simulink model "ControlSystem"  (R2021b)
settings: Solver=VariableStepAuto  StartTime=simIn(1,1)  StopTime=simIn(end,1)  RelTol=1e-3
values from neighbouring files (symbols this model uses):
  A = -inv(L)*R    [PlasmalessModel.m]
  B = L\S    [PlasmalessModel.m]
  C = eye(circuitNumber,length(A))    [PlasmalessModel.m]
  Controller = struct('R1',pid(Rcontr(1,1)),'R2',pid(Rcontr(2,2)),'R3',pid(Rcontr(3,3)),'R4',pid(Rcontr(4,4)),'R5',      pid(Rcontr(5,5)),'R6',pid(Rcontr(6,6)),'R7',pid(Rcontr(7,7)),'R8',pid(Rcontr(8,8)),'R9',pid(Rcontr(9,9)),'R10',      pid(Rcontr(10,10)),'R11',pid(Rcontr(11,11)),'R12',pid(Rcontr(12,12)))    [GeneticAlgorithm.m]    (also in OptimalTunedGA.mat = ; PIDController.m = struct('R1',R1,'R2',R2,'R3',R3,'R4',R4,'R5',R5,'R6',R6,     ; RLocusController.m = struct('R1',R1,'R2',R2,'R3',R3,'R4',R4,'R5',R5,'R6',R6,     )
  D = zeros(circuitNumber,circuitNumber)    [PlasmalessModel.m]
  dt = 0.001    [GeneticAlgorithm.m]    (also in PlasmalessModel.m; ReferenceDatabase.m)
  fil1 = zpk(minreal(R1 - k1 - r1(end)/s, 1e-2))    [RLocusController.m]
  fil10 = zpk(minreal(R10 - k10 - r10(end)/s, 1e-2))    [RLocusController.m]
  fil11 = zpk(minreal(R11 - k11 - r11(end)/s, 1e-2))    [RLocusController.m]
  fil12 = zpk(minreal(R12 - k12 - r12(end)/s, 1e-2))    [RLocusController.m]
  fil2 = zpk(minreal(R2 - k2 - r2(end)/s, 1e-2))    [RLocusController.m]
  fil3 = zpk(minreal(R3 - k3 - r3(end)/s, 1e-2))    [RLocusController.m]
  fil4 = zpk(minreal(R4 - k4 - r4(end)/s, 1e-2))    [RLocusController.m]
  fil5 = zpk(minreal(R5 - k5 - r5(end)/s, 1e-2))    [RLocusController.m]
  fil6 = zpk(minreal(R6 - k6 - r6(end)/s, 1e-2))    [RLocusController.m]
  fil7 = zpk(minreal(R7 - k7 - r7(end)/s, 1e-2))    [RLocusController.m]
  fil8 = zpk(minreal(R8 - k8 - r8(end)/s, 1e-2))    [RLocusController.m]
  fil9 = zpk(minreal(R9 - k9 - r9(end)/s, 1e-2))    [RLocusController.m]
  PSdelay = 1.67e-3    (= 0.00167)    [PlasmalessModel.m]
  PSden = [7e-3 1]    [PlasmalessModel.m]
  PSnum = 1    [PlasmalessModel.m]
  PSsat = [350 350 350 350 350 350           800 800 400 400 330 330]    [PlasmalessModel.m]
  sys1 = balred(sys(1,1),ord)    [PlasmalessModel.m]
  sys10 = balred(sys(10,10),ord)    [PlasmalessModel.m]
  sys11 = balred(sys(11,11),ord)    [PlasmalessModel.m]
  sys12 = balred(sys(12,12),ord)    [PlasmalessModel.m]
  sys2 = balred(sys(2,2),ord)    [PlasmalessModel.m]
  sys3 = balred(sys(3,3),ord)    [PlasmalessModel.m]
  sys4 = balred(sys(4,4),ord)    [PlasmalessModel.m]
  sys5 = balred(sys(5,5),ord)    [PlasmalessModel.m]
  sys6 = balred(sys(6,6),ord)    [PlasmalessModel.m]
  sys7 = balred(sys(7,7),ord)    [PlasmalessModel.m]
  sys8 = balred(sys(8,8),ord)    [PlasmalessModel.m]
  sys9 = balred(sys(9,9),ord)    [PlasmalessModel.m]
  varIpf = Scenario.Reference4.var    [PlasmalessModel.m]    (also in ReferenceDatabase.m)
undefined symbols (not defined in the file or in its folder): k1, k10, k11, k12, k2, k3, k4, k5, k6, k7, k8, k9
libraries: simulink x98, cstblocks x60
(part 2 of 4)

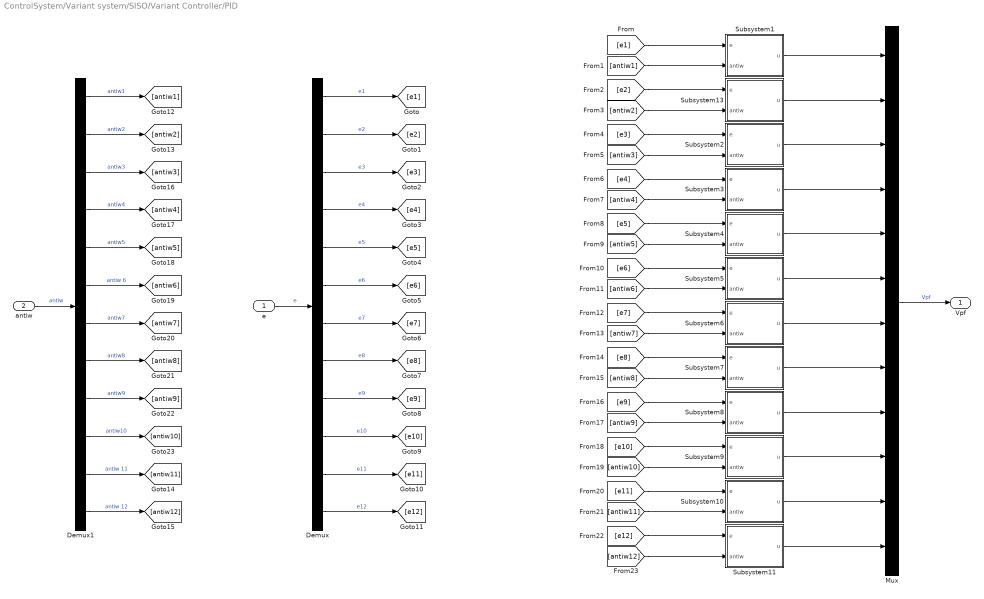
== system ControlSystem/Variant system/SISO/Variant Controller/PID ==
  e : Inport
  antiw : Inport  Port=2
  Demux : Demux  Outputs=12
  Demux1 : Demux  Outputs=12
  Mux : Mux  Inputs=12
  Subsystem1 : Subsystem  mask(Custom PID){Ki=Controller.R1.Ki, Kp=Controller.R1.Kp, Kd=Controller.R1.Kd, Tf=[Controller.R1.Tf 1], Threshold=PSsat(1)}
      mask prompts: Ki "Integral Gain"; Kp "Proportional Gain"; Kd "Derivative Gain"; Tf "Filtered Derivative"
      mask TypeOptions Ki: Integral Gain/Gain
      mask TypeOptions Kp: Proportional Gain/Gain
      mask TypeOptions Kd: Derivative Gain/Gain
      mask TypeOptions Tf: Filtered Derivative/Denominator
      mask TypeOptions Threshold:
      | Clamping/Compare
      | To Threshold/const
      mask DialogControl Container1 Prompt: Gain and Compensator
      mask DialogControl Container2 Prompt: Anti Windup
  Subsystem10 : Subsystem  mask(Custom PID){Ki=Controller.R11.Ki, Kp=Controller.R11.Kp, Kd=Controller.R11.Kd, Tf=[Controller.R11.Tf 1], Threshold=PSsat(11)}
      mask prompts: Ki "Integral Gain"; Kp "Proportional Gain"; Kd "Derivative Gain"; Tf "Filtered Derivative"
      mask TypeOptions Ki: Integral Gain/Gain
      mask TypeOptions Kp: Proportional Gain/Gain
      mask TypeOptions Kd: Derivative Gain/Gain
      mask TypeOptions Tf: Filtered Derivative/Denominator
      mask TypeOptions Threshold:
      | Clamping/Compare
      | To Threshold/const
      mask DialogControl Container1 Prompt: Gain and Compensator
      mask DialogControl Container2 Prompt: Anti Windup
  Subsystem11 : Subsystem  mask(Custom PID){Ki=Controller.R12.Ki, Kp=Controller.R12.Kp, Kd=Controller.R12.Kd, Tf=[Controller.R12.Tf 1], Threshold=PSsat(12)}
      mask prompts: Ki "Integral Gain"; Kp "Proportional Gain"; Kd "Derivative Gain"; Tf "Filtered Derivative"
      mask TypeOptions Ki: Integral Gain/Gain
      mask TypeOptions Kp: Proportional Gain/Gain
      mask TypeOptions Kd: Derivative Gain/Gain
      mask TypeOptions Tf: Filtered Derivative/Denominator
      mask TypeOptions Threshold:
      | Clamping/Compare
      | To Threshold/const
      mask DialogControl Container1 Prompt: Gain and Compensator
      mask DialogControl Container2 Prompt: Anti Windup
  Subsystem13 : Subsystem  mask(Custom PID){Ki=Controller.R2.Ki, Kp=Controller.R2.Kp, Kd=Controller.R2.Kd, Tf=[Controller.R2.Tf 1], Threshold=PSsat(2)}
      mask prompts: Ki "Integral Gain"; Kp "Proportional Gain"; Kd "Derivative Gain"; Tf "Filtered Derivative"
      mask TypeOptions Ki: Integral Gain/Gain
      mask TypeOptions Kp: Proportional Gain/Gain
      mask TypeOptions Kd: Derivative Gain/Gain
      mask TypeOptions Tf: Filtered Derivative/Denominator
      mask TypeOptions Threshold:
      | Clamping/Compare
      | To Threshold/const
      mask DialogControl Container1 Prompt: Gain and Compensator
      mask DialogControl Container2 Prompt: Anti Windup
  Subsystem2 : Subsystem  mask(Custom PID){Ki=Controller.R3.Ki, Kp=Controller.R3.Kp, Kd=Controller.R3.Kd, Tf=[Controller.R3.Tf 1], Threshold=PSsat(3)}
      mask prompts: Ki "Integral Gain"; Kp "Proportional Gain"; Kd "Derivative Gain"; Tf "Filtered Derivative"
      mask TypeOptions Ki: Integral Gain/Gain
      mask TypeOptions Kp: Proportional Gain/Gain
      mask TypeOptions Kd: Derivative Gain/Gain
      mask TypeOptions Tf: Filtered Derivative/Denominator
      mask TypeOptions Threshold:
      | Clamping/Compare
      | To Threshold/const
      mask DialogControl Container1 Prompt: Gain and Compensator
      mask DialogControl Container2 Prompt: Anti Windup
  Subsystem3 : Subsystem  mask(Custom PID){Ki=Controller.R4.Ki, Kp=Controller.R4.Kp, Kd=Controller.R4.Kd, Tf=[Controller.R4.Tf 1], Threshold=PSsat(4)}
      mask prompts: Ki "Integral Gain"; Kp "Proportional Gain"; Kd "Derivative Gain"; Tf "Filtered Derivative"
      mask TypeOptions Ki: Integral Gain/Gain
      mask TypeOptions Kp: Proportional Gain/Gain
      mask TypeOptions Kd: Derivative Gain/Gain
      mask TypeOptions Tf: Filtered Derivative/Denominator
      mask TypeOptions Threshold:
      | Clamping/Compare
      | To Threshold/const
      mask DialogControl Container1 Prompt: Gain and Compensator
      mask DialogControl Container2 Prompt: Anti Windup
  Subsystem4 : Subsystem  mask(Custom PID){Ki=Controller.R5.Ki, Kp=Controller.R5.Kp, Kd=Controller.R5.Kd, Tf=[Controller.R5.Tf 1], Threshold=PSsat(5)}
      mask prompts: Ki "Integral Gain"; Kp "Proportional Gain"; Kd "Derivative Gain"; Tf "Filtered Derivative"
      mask TypeOptions Ki: Integral Gain/Gain
      mask TypeOptions Kp: Proportional Gain/Gain
      mask TypeOptions Kd: Derivative Gain/Gain
      mask TypeOptions Tf: Filtered Derivative/Denominator
      mask TypeOptions Threshold:
      | Clamping/Compare
      | To Threshold/const
      mask DialogControl Container1 Prompt: Gain and Compensator
      mask DialogControl Container2 Prompt: Anti Windup
  Subsystem5 : Subsystem  mask(Custom PID){Ki=Controller.R6.Ki, Kp=Controller.R6.Kp, Kd=Controller.R6.Kd, Tf=[Controller.R6.Tf 1], Threshold=PSsat(6)}
      mask prompts: Ki "Integral Gain"; Kp "Proportional Gain"; Kd "Derivative Gain"; Tf "Filtered Derivative"
      mask TypeOptions Ki: Integral Gain/Gain
      mask TypeOptions Kp: Proportional Gain/Gain
      mask TypeOptions Kd: Derivative Gain/Gain
      mask TypeOptions Tf: Filtered Derivative/Denominator
      mask TypeOptions Threshold:
      | Clamping/Compare
      | To Threshold/const
      mask DialogControl Container1 Prompt: Gain and Compensator
      mask DialogControl Container2 Prompt: Anti Windup
  Subsystem6 : Subsystem  mask(Custom PID){Ki=Controller.R7.Ki, Kp=Controller.R7.Kp, Kd=Controller.R7.Kd, Tf=[Controller.R7.Tf 1], Threshold=PSsat(7)}
      mask prompts: Ki "Integral Gain"; Kp "Proportional Gain"; Kd "Derivative Gain"; Tf "Filtered Derivative"
      mask TypeOptions Ki: Integral Gain/Gain
      mask TypeOptions Kp: Proportional Gain/Gain
      mask TypeOptions Kd: Derivative Gain/Gain
      mask TypeOptions Tf: Filtered Derivative/Denominator
      mask TypeOptions Threshold:
      | Clamping/Compare
      | To Threshold/const
      mask DialogControl Container1 Prompt: Gain and Compensator
      mask DialogControl Container2 Prompt: Anti Windup
  Subsystem7 : Subsystem  mask(Custom PID){Ki=Controller.R8.Ki, Kp=Controller.R8.Kp, Kd=Controller.R8.Kd, Tf=[Controller.R8.Tf 1], Threshold=PSsat(8)}
      mask prompts: Ki "Integral Gain"; Kp "Proportional Gain"; Kd "Derivative Gain"; Tf "Filtered Derivative"
      mask TypeOptions Ki: Integral Gain/Gain
      mask TypeOptions Kp: Proportional Gain/Gain
      mask TypeOptions Kd: Derivative Gain/Gain
      mask TypeOptions Tf: Filtered Derivative/Denominator
      mask TypeOptions Threshold:
      | Clamping/Compare
      | To Threshold/const
      mask DialogControl Container1 Prompt: Gain and Compensator
      mask DialogControl Container2 Prompt: Anti Windup
  Subsystem8 : Subsystem  mask(Custom PID){Ki=Controller.R9.Ki, Kp=Controller.R9.Kp, Kd=Controller.R9.Kd, Tf=[Controller.R9.Tf 1], Threshold=PSsat(9)}
      mask prompts: Ki "Integral Gain"; Kp "Proportional Gain"; Kd "Derivative Gain"; Tf "Filtered Derivative"
      mask TypeOptions Ki: Integral Gain/Gain
      mask TypeOptions Kp: Proportional Gain/Gain
      mask TypeOptions Kd: Derivative Gain/Gain
      mask TypeOptions Tf: Filtered Derivative/Denominator
      mask TypeOptions Threshold:
      | Clamping/Compare
      | To Threshold/const
      mask DialogControl Container1 Prompt: Gain and Compensator
      mask DialogControl Container2 Prompt: Anti Windup
  Subsystem9 : Subsystem  mask(Custom PID){Ki=Controller.R10.Ki, Kp=Controller.R10.Kp, Kd=Controller.R10.Kd, Tf=[Controller.R10.Tf 1], Threshold=PSsat(10)}
      mask prompts: Ki "Integral Gain"; Kp "Proportional Gain"; Kd "Derivative Gain"; Tf "Filtered Derivative"
      mask TypeOptions Ki: Integral Gain/Gain
      mask TypeOptions Kp: Proportional Gain/Gain
      mask TypeOptions Kd: Derivative Gain/Gain
      mask TypeOptions Tf: Filtered Derivative/Denominator
      mask TypeOptions Threshold:
      | Clamping/Compare
      | To Threshold/const
      mask DialogControl Container1 Prompt: Gain and Compensator
      mask DialogControl Container2 Prompt: Anti Windup
  Vpf : Outport
  wires:
  Subsystem10/1(u) -> Mux/11
  e/1 -> Demux/1  "e"
  [antiw3] -> Subsystem2/2(antiw)
  Demux/1 -> [e1]  "e1"
  [e1] -> Subsystem1/1(e)
  Demux1/7 -> [antiw7]  "antiw7"
  Demux/2 -> [e2]  "e2"
  Demux/12 -> [e12]  "e12"
  Subsystem8/1(u) -> Mux/9
  Demux/3 -> [e3]  "e3"
  Demux/8 -> [e8]  "e8"
  Demux/9 -> [e9]  "e9"
  Demux1/2 -> [antiw2]  "antiw2"
  Demux/7 -> [e7]  "e7"
  Demux1/1 -> [antiw1]  "antiw1"
  Demux/11 -> [e11]  "e11"
  Demux1/5 -> [antiw5]  "antiw5"
  [e6] -> Subsystem5/1(e)
  [antiw7] -> Subsystem6/2(antiw)
  [e11] -> Subsystem10/1(e)
  [e5] -> Subsystem4/1(e)
  [e12] -> Subsystem11/1(e)
  Demux1/10 -> [antiw10]  "antiw10"
  [antiw4] -> Subsystem3/2(antiw)
  Demux1/8 -> [antiw8]  "antiw8"
  [antiw6] -> Subsystem5/2(antiw)
  [e10] -> Subsystem9/1(e)
  [antiw11] -> Subsystem10/2(antiw)
  antiw/1 -> Demux1/1  "antiw"
  Demux/6 -> [e6]  "e6"
  Demux1/11 -> [antiw11]  "antiw 11"
  [e3] -> Subsystem2/1(e)
  Demux1/6 -> [antiw6]  "antiw 6"
  Demux1/3 -> [antiw3]  "antiw3"
  Demux1/12 -> [antiw12]  "antiw 12"
  [e9] -> Subsystem8/1(e)
  [antiw2] -> Subsystem13/2(antiw)
  Demux1/9 -> [antiw9]  "antiw9"
  [antiw10] -> Subsystem9/2(antiw)
  [antiw8] -> Subsystem7/2(antiw)
  Subsystem3/1(u) -> Mux/4
  Demux/10 -> [e10]  "e10"
  Demux/5 -> [e5]  "e5"
  Subsystem2/1(u) -> Mux/3
  Demux/4 -> [e4]  "e4"
  Subsystem5/1(u) -> Mux/6
  [antiw9] -> Subsystem8/2(antiw)
  Subsystem1/1(u) -> Mux/1
  Mux/1 -> Vpf/1  "Vpf"
  Subsystem11/1(u) -> Mux/12
  [antiw1] -> Subsystem1/2(antiw)
  [antiw5] -> Subsystem4/2(antiw)
  [antiw12] -> Subsystem11/2(antiw)
  [e7] -> Subsystem6/1(e)
  Subsystem13/1(u) -> Mux/2
  [e4] -> Subsystem3/1(e)
  Demux1/4 -> [antiw4]  "antiw4"
  [e8] -> Subsystem7/1(e)
  Subsystem6/1(u) -> Mux/7
  Subsystem7/1(u) -> Mux/8
  Subsystem9/1(u) -> Mux/10
  Subsystem4/1(u) -> Mux/5
  [e2] -> Subsystem13/1(e)

== system ControlSystem/Variant system/SISO/Variant Controller/RlocusNOantiwindup ==
  e : Inport
  Demux : Demux  Outputs=12
  LTI System : cstblocks/LTI System  sys=R1  IC=[]
  LTI System1 : cstblocks/LTI System  sys=R2  IC=[]
  LTI System10 : cstblocks/LTI System  sys=R11  IC=[]
  LTI System11 : cstblocks/LTI System  sys=R12  IC=[]
  LTI System2 : cstblocks/LTI System  sys=R3  IC=[]
  LTI System3 : cstblocks/LTI System  sys=R4  IC=[]
  LTI System4 : cstblocks/LTI System  sys=R5  IC=[]
  LTI System5 : cstblocks/LTI System  sys=R6  IC=[]
  LTI System6 : cstblocks/LTI System  sys=R7  IC=[]
  LTI System7 : cstblocks/LTI System  sys=R8  IC=[]
  LTI System8 : cstblocks/LTI System  sys=R9  IC=[]
  LTI System9 : cstblocks/LTI System  sys=R10  IC=[]
  Mux : Mux  Inputs=12
  Vpf : Outport
  wires:
  LTI System11/1 -> Mux/12
  LTI System1/1 -> Mux/2
  LTI System5/1 -> Mux/6
  LTI System7/1 -> Mux/8
  Demux/10 -> LTI System9/1
  Demux/8 -> LTI System7/1
  Demux/7 -> LTI System6/1
  Demux/6 -> LTI System5/1
  LTI System/1 -> Mux/1
  Demux/12 -> LTI System11/1
  Demux/3 -> LTI System2/1
  Demux/1 -> LTI System/1
  LTI System2/1 -> Mux/3
  Demux/4 -> LTI System3/1
  LTI System4/1 -> Mux/5
  Demux/2 -> LTI System1/1
  Demux/9 -> LTI System8/1
  Demux/5 -> LTI System4/1
  LTI System3/1 -> Mux/4
  LTI System10/1 -> Mux/11
  LTI System6/1 -> Mux/7
  e/1 -> Demux/1  "e"
  Mux/1 -> Vpf/1  "Vpf"
  LTI System8/1 -> Mux/9
  LTI System9/1 -> Mux/10
  Demux/11 -> LTI System10/1

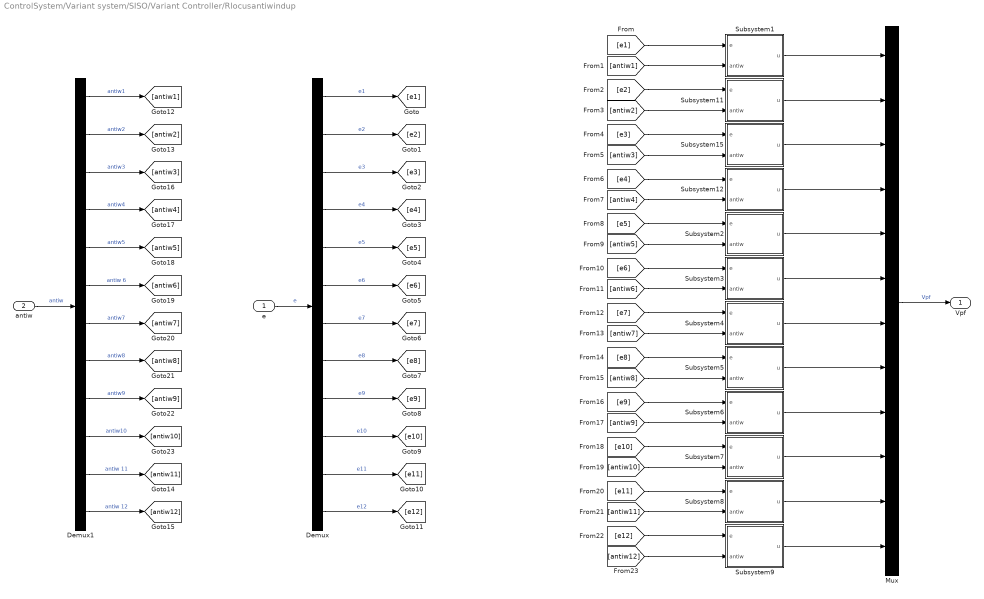
== system ControlSystem/Variant system/SISO/Variant Controller/Rlocusantiwindup ==
  e : Inport
  antiw : Inport  Port=2
  Demux : Demux  Outputs=12
  Demux1 : Demux  Outputs=12
  Mux : Mux  Inputs=12
  Subsystem1 : Subsystem  mask(Fractal Transfer Function){Ki=r1(end), Kp=k1, Compensator=fil1, Threshold=PSsat(1)}
      mask prompts: Ki "Integral Gain"; Kp "Proportional Gain"
      mask help: Fractal Transfer Function of a controller in a general rational transfer function form. The controller is decomposed in an Integral term, a Proportional term and a compensator.
      mask TypeOptions Ki: Integral Gain/Gain
      mask TypeOptions Kp: Proportional Gain/Gain
      mask TypeOptions Compensator: ZPK compensator/sys
      mask TypeOptions Threshold:
      | Clamping/Compare
      | To Threshold/const
      mask DialogControl Container1 Prompt: Gain and Compensator
      mask DialogControl Container2 Prompt: Anti Windup
  Subsystem11 : Subsystem  mask(Fractal Transfer Function){Ki=r2(end), Kp=k2, Compensator=fil2, Threshold=PSsat(2)}
      mask prompts: Ki "Integral Gain"; Kp "Proportional Gain"
      mask help: Fractal Transfer Function of a controller in a general rational transfer function form. The controller is decomposed in an Integral term, a Proportional term and a compensator.
      mask TypeOptions Ki: Integral Gain/Gain
      mask TypeOptions Kp: Proportional Gain/Gain
      mask TypeOptions Compensator: ZPK compensator/sys
      mask TypeOptions Threshold:
      | Clamping/Compare
      | To Threshold/const
      mask DialogControl Container1 Prompt: Gain and Compensator
      mask DialogControl Container2 Prompt: Anti Windup
  Subsystem12 : Subsystem  mask(Fractal Transfer Function){Ki=r4(end), Kp=k4, Compensator=fil4, Threshold=PSsat(4)}
      mask prompts: Ki "Integral Gain"; Kp "Proportional Gain"
      mask help: Fractal Transfer Function of a controller in a general rational transfer function form. The controller is decomposed in an Integral term, a Proportional term and a compensator.
      mask TypeOptions Ki: Integral Gain/Gain
      mask TypeOptions Kp: Proportional Gain/Gain
      mask TypeOptions Compensator: ZPK compensator/sys
      mask TypeOptions Threshold:
      | Clamping/Compare
      | To Threshold/const
      mask DialogControl Container1 Prompt: Gain and Compensator
      mask DialogControl Container2 Prompt: Anti Windup
  Subsystem15 : Subsystem  mask(Fractal Transfer Function){Ki=r3(end), Kp=k3, Compensator=fil3, Threshold=PSsat(3)}
      mask prompts: Ki "Integral Gain"; Kp "Proportional Gain"
      mask help: Fractal Transfer Function of a controller in a general rational transfer function form. The controller is decomposed in an Integral term, a Proportional term and a compensator.
      mask TypeOptions Ki: Integral Gain/Gain
      mask TypeOptions Kp: Proportional Gain/Gain
      mask TypeOptions Compensator: ZPK compensator/sys
      mask TypeOptions Threshold:
      | Clamping/Compare
      | To Threshold/const
      mask DialogControl Container1 Prompt: Gain and Compensator
      mask DialogControl Container2 Prompt: Anti Windup
  Subsystem2 : Subsystem  mask(Fractal Transfer Function){Ki=r5(end), Kp=k5, Compensator=fil5, Threshold=PSsat(5)}
      mask prompts: Ki "Integral Gain"; Kp "Proportional Gain"
      mask help: Fractal Transfer Function of a controller in a general rational transfer function form. The controller is decomposed in an Integral term, a Proportional term and a compensator.
      mask TypeOptions Ki: Integral Gain/Gain
      mask TypeOptions Kp: Proportional Gain/Gain
      mask TypeOptions Compensator: ZPK compensator/sys
      mask TypeOptions Threshold:
      | Clamping/Compare
      | To Threshold/const
      mask DialogControl Container1 Prompt: Gain and Compensator
      mask DialogControl Container2 Prompt: Anti Windup
  Subsystem3 : Subsystem  mask(Fractal Transfer Function){Ki=r6(end), Kp=k6, Compensator=fil6, Threshold=PSsat(6)}
      mask prompts: Ki "Integral Gain"; Kp "Proportional Gain"
      mask help: Fractal Transfer Function of a controller in a general rational transfer function form. The controller is decomposed in an Integral term, a Proportional term and a compensator.
      mask TypeOptions Ki: Integral Gain/Gain
      mask TypeOptions Kp: Proportional Gain/Gain
      mask TypeOptions Compensator: ZPK compensator/sys
      mask TypeOptions Threshold:
      | Clamping/Compare
      | To Threshold/const
      mask DialogControl Container1 Prompt: Gain and Compensator
      mask DialogControl Container2 Prompt: Anti Windup
  Subsystem4 : Subsystem  mask(Fractal Transfer Function){Ki=r7(end), Kp=k7, Compensator=fil7, Threshold=PSsat(7)}
      mask prompts: Ki "Integral Gain"; Kp "Proportional Gain"
      mask help: Fractal Transfer Function of a controller in a general rational transfer function form. The controller is decomposed in an Integral term, a Proportional term and a compensator.
      mask TypeOptions Ki: Integral Gain/Gain
      mask TypeOptions Kp: Proportional Gain/Gain
      mask TypeOptions Compensator: ZPK compensator/sys
      mask TypeOptions Threshold:
      | Clamping/Compare
      | To Threshold/const
      mask DialogControl Container1 Prompt: Gain and Compensator
      mask DialogControl Container2 Prompt: Anti Windup
  Subsystem5 : Subsystem  mask(Fractal Transfer Function){Ki=r8(end), Kp=k8, Compensator=fil8, Threshold=PSsat(8)}
      mask prompts: Ki "Integral Gain"; Kp "Proportional Gain"
      mask help: Fractal Transfer Function of a controller in a general rational transfer function form. The controller is decomposed in an Integral term, a Proportional term and a compensator.
      mask TypeOptions Ki: Integral Gain/Gain
      mask TypeOptions Kp: Proportional Gain/Gain
      mask TypeOptions Compensator: ZPK compensator/sys
      mask TypeOptions Threshold:
      | Clamping/Compare
      | To Threshold/const
      mask DialogControl Container1 Prompt: Gain and Compensator
      mask DialogControl Container2 Prompt: Anti Windup
  Subsystem6 : Subsystem  mask(Fractal Transfer Function){Ki=r9(end), Kp=k9, Compensator=fil9, Threshold=PSsat(9)}
      mask prompts: Ki "Integral Gain"; Kp "Proportional Gain"
      mask help: Fractal Transfer Function of a controller in a general rational transfer function form. The controller is decomposed in an Integral term, a Proportional term and a compensator.
      mask TypeOptions Ki: Integral Gain/Gain
      mask TypeOptions Kp: Proportional Gain/Gain
      mask TypeOptions Compensator: ZPK compensator/sys
      mask TypeOptions Threshold:
      | Clamping/Compare
      | To Threshold/const
      mask DialogControl Container1 Prompt: Gain and Compensator
      mask DialogControl Container2 Prompt: Anti Windup
  Subsystem7 : Subsystem  mask(Fractal Transfer Function){Ki=r10(end), Kp=k10, Compensator=fil10, Threshold=PSsat(10)}
      mask prompts: Ki "Integral Gain"; Kp "Proportional Gain"
      mask help: Fractal Transfer Function of a controller in a general rational transfer function form. The controller is decomposed in an Integral term, a Proportional term and a compensator.
      mask TypeOptions Ki: Integral Gain/Gain
      mask TypeOptions Kp: Proportional Gain/Gain
      mask TypeOptions Compensator: ZPK compensator/sys
      mask TypeOptions Threshold:
      | Clamping/Compare
      | To Threshold/const
      mask DialogControl Container1 Prompt: Gain and Compensator
      mask DialogControl Container2 Prompt: Anti Windup
  Subsystem8 : Subsystem  mask(Fractal Transfer Function){Ki=r11(end), Kp=k11, Compensator=fil11, Threshold=PSsat(11)}
      mask prompts: Ki "Integral Gain"; Kp "Proportional Gain"
      mask help: Fractal Transfer Function of a controller in a general rational transfer function form. The controller is decomposed in an Integral term, a Proportional term and a compensator.
      mask TypeOptions Ki: Integral Gain/Gain
      mask TypeOptions Kp: Proportional Gain/Gain
      mask TypeOptions Compensator: ZPK compensator/sys
      mask TypeOptions Threshold:
      | Clamping/Compare
      | To Threshold/const
      mask DialogControl Container1 Prompt: Gain and Compensator
      mask DialogControl Container2 Prompt: Anti Windup
  Subsystem9 : Subsystem  mask(Fractal Transfer Function){Ki=r12(end), Kp=k12, Compensator=fil12, Threshold=PSsat(12)}
      mask prompts: Ki "Integral Gain"; Kp "Proportional Gain"
      mask help: Fractal Transfer Function of a controller in a general rational transfer function form. The controller is decomposed in an Integral term, a Proportional term and a compensator.
      mask TypeOptions Ki: Integral Gain/Gain
      mask TypeOptions Kp: Proportional Gain/Gain
      mask TypeOptions Compensator: ZPK compensator/sys
      mask TypeOptions Threshold:
      | Clamping/Compare
      | To Threshold/const
      mask DialogControl Container1 Prompt: Gain and Compensator
      mask DialogControl Container2 Prompt: Anti Windup
  Vpf : Outport
  wires:
  [e2] -> Subsystem11/1(e)
  Subsystem2/1(u) -> Mux/5
  Subsystem7/1(u) -> Mux/10
  Subsystem5/1(u) -> Mux/8
  Subsystem4/1(u) -> Mux/7
  [e8] -> Subsystem5/1(e)
  Demux1/4 -> [antiw4]  "antiw4"
  [e4] -> Subsystem12/1(e)
  Subsystem11/1(u) -> Mux/2
  [e7] -> Subsystem4/1(e)
  [antiw12] -> Subsystem9/2(antiw)
  [antiw5] -> Subsystem2/2(antiw)
  [antiw1] -> Subsystem1/2(antiw)
  Subsystem9/1(u) -> Mux/12
  Mux/1 -> Vpf/1  "Vpf"
  Subsystem1/1(u) -> Mux/1
  [antiw9] -> Subsystem6/2(antiw)
  Subsystem3/1(u) -> Mux/6
  Demux/4 -> [e4]  "e4"
  Subsystem15/1(u) -> Mux/3
  Demux/5 -> [e5]  "e5"
  Demux/10 -> [e10]  "e10"
  Subsystem12/1(u) -> Mux/4
  [antiw8] -> Subsystem5/2(antiw)
  [antiw10] -> Subsystem7/2(antiw)
  Demux1/9 -> [antiw9]  "antiw9"
  [antiw2] -> Subsystem11/2(antiw)
  [e9] -> Subsystem6/1(e)
  Demux1/12 -> [antiw12]  "antiw 12"
  Demux1/3 -> [antiw3]  "antiw3"
  Demux1/6 -> [antiw6]  "antiw 6"
  [e3] -> Subsystem15/1(e)
  Demux1/11 -> [antiw11]  "antiw 11"
  Demux/6 -> [e6]  "e6"
  antiw/1 -> Demux1/1  "antiw"
  [antiw11] -> Subsystem8/2(antiw)
  [e10] -> Subsystem7/1(e)
  [antiw6] -> Subsystem3/2(antiw)
  Demux1/8 -> [antiw8]  "antiw8"
  [antiw4] -> Subsystem12/2(antiw)
  Demux1/10 -> [antiw10]  "antiw10"
  [e12] -> Subsystem9/1(e)
  [e5] -> Subsystem2/1(e)
  [e11] -> Subsystem8/1(e)
  [antiw7] -> Subsystem4/2(antiw)
  [e6] -> Subsystem3/1(e)
  Demux1/5 -> [antiw5]  "antiw5"
  Demux/11 -> [e11]  "e11"
  Demux1/1 -> [antiw1]  "antiw1"
  Demux/7 -> [e7]  "e7"
  Demux1/2 -> [antiw2]  "antiw2"
  Demux/9 -> [e9]  "e9"
  Demux/8 -> [e8]  "e8"
  Demux/3 -> [e3]  "e3"
  Subsystem6/1(u) -> Mux/9
  Demux/12 -> [e12]  "e12"
  Demux/2 -> [e2]  "e2"
  Demux1/7 -> [antiw7]  "antiw7"
  [e1] -> Subsystem1/1(e)
  Demux/1 -> [e1]  "e1"
  [antiw3] -> Subsystem15/2(antiw)
  e/1 -> Demux/1  "e"
  Subsystem8/1(u) -> Mux/11

== system ControlSystem/Variant system/MIMO/Variant Controller/PID/Subsystem1 ==
  e : Inport
  antiw : Inport  Port=2
  Avoid windup : Constant  Value=0
  Clamping : Subsystem
  Derivative Gain : Gain  Gain=Kd
  Filtered Derivative : TransferFcn  Denominator=Tf
  Integral Gain : Gain  Gain=Ki
  Integrator : Integrator
  Proportional Gain : Gain  Gain=Kp
  Sum action : Sum  Inputs=+++
  Switch1 : Switch  Criteria=u2 > Threshold
  u : Outport
  wires:
  Clamping/1(Clamping) -> Switch1/2  "Clamping"
  antiw/1 -> Clamping/2(antiw)  "antiw"
  Integrator/1 -> Sum action/3
  Proportional Gain/1 -> Sum action/1
  Avoid windup/1 -> Switch1/1
  Integral Gain/1 -> Switch1/3
  Switch1/1 -> Integrator/1
  e/1 -> Derivative Gain/1, Integral Gain/1, Clamping/3(e), Proportional Gain/1  "e"
  Derivative Gain/1 -> Filtered Derivative/1
  Sum action/1 -> u/1, Clamping/1(u)  "u"
  Filtered Derivative/1 -> Sum action/2

== system ControlSystem/Variant system/MIMO/Variant Controller/PID/Subsystem10 ==
  e : Inport
  antiw : Inport  Port=2
  Avoid windup : Constant  Value=0
  Clamping : Subsystem
  Derivative Gain : Gain  Gain=Kd
  Filtered Derivative : TransferFcn  Denominator=Tf
  Integral Gain : Gain  Gain=Ki
  Integrator : Integrator
  Proportional Gain : Gain  Gain=Kp
  Sum action : Sum  Inputs=+++
  Switch1 : Switch  Criteria=u2 > Threshold
  u : Outport
  wires:
  Clamping/1(Clamping) -> Switch1/2  "Clamping"
  antiw/1 -> Clamping/2(antiw)  "antiw"
  Integrator/1 -> Sum action/3
  Proportional Gain/1 -> Sum action/1
  Avoid windup/1 -> Switch1/1
  Integral Gain/1 -> Switch1/3
  Switch1/1 -> Integrator/1
  e/1 -> Derivative Gain/1, Integral Gain/1, Clamping/3(e), Proportional Gain/1  "e"
  Derivative Gain/1 -> Filtered Derivative/1
  Sum action/1 -> u/1, Clamping/1(u)  "u"
  Filtered Derivative/1 -> Sum action/2

== system ControlSystem/Variant system/MIMO/Variant Controller/PID/Subsystem11 ==
  e : Inport
  antiw : Inport  Port=2
  Avoid windup : Constant  Value=0
  Clamping : Subsystem
  Derivative Gain : Gain  Gain=Kd
  Filtered Derivative : TransferFcn  Denominator=Tf
  Integral Gain : Gain  Gain=Ki
  Integrator : Integrator
  Proportional Gain : Gain  Gain=Kp
  Sum action : Sum  Inputs=+++
  Switch1 : Switch  Criteria=u2 > Threshold
  u : Outport
  wires:
  Filtered Derivative/1 -> Sum action/2
  Sum action/1 -> Clamping/1(u), u/1  "u"
  Derivative Gain/1 -> Filtered Derivative/1
  e/1 -> Proportional Gain/1, Clamping/3(e), Integral Gain/1, Derivative Gain/1  "e"
  Switch1/1 -> Integrator/1
  Integral Gain/1 -> Switch1/3
  Avoid windup/1 -> Switch1/1
  Proportional Gain/1 -> Sum action/1
  Integrator/1 -> Sum action/3
  antiw/1 -> Clamping/2(antiw)  "antiw"
  Clamping/1(Clamping) -> Switch1/2  "Clamping"

== system ControlSystem/Variant system/MIMO/Variant Controller/PID/Subsystem13 ==
  e : Inport
  antiw : Inport  Port=2
  Avoid windup : Constant  Value=0
  Clamping : Subsystem
  Derivative Gain : Gain  Gain=Kd
  Filtered Derivative : TransferFcn  Denominator=Tf
  Integral Gain : Gain  Gain=Ki
  Integrator : Integrator
  Proportional Gain : Gain  Gain=Kp
  Sum action : Sum  Inputs=+++
  Switch1 : Switch  Criteria=u2 > Threshold
  u : Outport
  wires:
  Filtered Derivative/1 -> Sum action/2
  Sum action/1 -> Clamping/1(u), u/1  "u"
  Derivative Gain/1 -> Filtered Derivative/1
  e/1 -> Proportional Gain/1, Clamping/3(e), Integral Gain/1, Derivative Gain/1  "e"
  Switch1/1 -> Integrator/1
  Integral Gain/1 -> Switch1/3
  Avoid windup/1 -> Switch1/1
  Proportional Gain/1 -> Sum action/1
  Integrator/1 -> Sum action/3
  antiw/1 -> Clamping/2(antiw)  "antiw"
  Clamping/1(Clamping) -> Switch1/2  "Clamping"

== system ControlSystem/Variant system/MIMO/Variant Controller/PID/Subsystem2 ==
  e : Inport
  antiw : Inport  Port=2
  Avoid windup : Constant  Value=0
  Clamping : Subsystem
  Derivative Gain : Gain  Gain=Kd
  Filtered Derivative : TransferFcn  Denominator=Tf
  Integral Gain : Gain  Gain=Ki
  Integrator : Integrator
  Proportional Gain : Gain  Gain=Kp
  Sum action : Sum  Inputs=+++
  Switch1 : Switch  Criteria=u2 > Threshold
  u : Outport
  wires:
  Clamping/1(Clamping) -> Switch1/2  "Clamping"
  antiw/1 -> Clamping/2(antiw)  "antiw"
  Integrator/1 -> Sum action/3
  Proportional Gain/1 -> Sum action/1
  Avoid windup/1 -> Switch1/1
  Integral Gain/1 -> Switch1/3
  Switch1/1 -> Integrator/1
  e/1 -> Derivative Gain/1, Integral Gain/1, Clamping/3(e), Proportional Gain/1  "e"
  Derivative Gain/1 -> Filtered Derivative/1
  Sum action/1 -> u/1, Clamping/1(u)  "u"
  Filtered Derivative/1 -> Sum action/2

== system ControlSystem/Variant system/MIMO/Variant Controller/PID/Subsystem3 ==
  e : Inport
  antiw : Inport  Port=2
  Avoid windup : Constant  Value=0
  Clamping : Subsystem
  Derivative Gain : Gain  Gain=Kd
  Filtered Derivative : TransferFcn  Denominator=Tf
  Integral Gain : Gain  Gain=Ki
  Integrator : Integrator
  Proportional Gain : Gain  Gain=Kp
  Sum action : Sum  Inputs=+++
  Switch1 : Switch  Criteria=u2 > Threshold
  u : Outport
  wires:
  Filtered Derivative/1 -> Sum action/2
  Sum action/1 -> Clamping/1(u), u/1  "u"
  Derivative Gain/1 -> Filtered Derivative/1
  e/1 -> Proportional Gain/1, Clamping/3(e), Integral Gain/1, Derivative Gain/1  "e"
  Switch1/1 -> Integrator/1
  Integral Gain/1 -> Switch1/3
  Avoid windup/1 -> Switch1/1
  Proportional Gain/1 -> Sum action/1
  Integrator/1 -> Sum action/3
  antiw/1 -> Clamping/2(antiw)  "antiw"
  Clamping/1(Clamping) -> Switch1/2  "Clamping"

== system ControlSystem/Variant system/MIMO/Variant Controller/PID/Subsystem4 ==
  e : Inport
  antiw : Inport  Port=2
  Avoid windup : Constant  Value=0
  Clamping : Subsystem
  Derivative Gain : Gain  Gain=Kd
  Filtered Derivative : TransferFcn  Denominator=Tf
  Integral Gain : Gain  Gain=Ki
  Integrator : Integrator
  Proportional Gain : Gain  Gain=Kp
  Sum action : Sum  Inputs=+++
  Switch1 : Switch  Criteria=u2 > Threshold
  u : Outport
  wires:
  Clamping/1(Clamping) -> Switch1/2  "Clamping"
  antiw/1 -> Clamping/2(antiw)  "antiw"
  Integrator/1 -> Sum action/3
  Proportional Gain/1 -> Sum action/1
  Avoid windup/1 -> Switch1/1
  Integral Gain/1 -> Switch1/3
  Switch1/1 -> Integrator/1
  e/1 -> Derivative Gain/1, Integral Gain/1, Clamping/3(e), Proportional Gain/1  "e"
  Derivative Gain/1 -> Filtered Derivative/1
  Sum action/1 -> u/1, Clamping/1(u)  "u"
  Filtered Derivative/1 -> Sum action/2

== system ControlSystem/Variant system/MIMO/Variant Controller/PID/Subsystem5 ==
  e : Inport
  antiw : Inport  Port=2
  Avoid windup : Constant  Value=0
  Clamping : Subsystem
  Derivative Gain : Gain  Gain=Kd
  Filtered Derivative : TransferFcn  Denominator=Tf
  Integral Gain : Gain  Gain=Ki
  Integrator : Integrator
  Proportional Gain : Gain  Gain=Kp
  Sum action : Sum  Inputs=+++
  Switch1 : Switch  Criteria=u2 > Threshold
  u : Outport
  wires:
  Filtered Derivative/1 -> Sum action/2
  Sum action/1 -> Clamping/1(u), u/1  "u"
  Derivative Gain/1 -> Filtered Derivative/1
  e/1 -> Proportional Gain/1, Clamping/3(e), Integral Gain/1, Derivative Gain/1  "e"
  Switch1/1 -> Integrator/1
  Integral Gain/1 -> Switch1/3
  Avoid windup/1 -> Switch1/1
  Proportional Gain/1 -> Sum action/1
  Integrator/1 -> Sum action/3
  antiw/1 -> Clamping/2(antiw)  "antiw"
  Clamping/1(Clamping) -> Switch1/2  "Clamping"

== system ControlSystem/Variant system/MIMO/Variant Controller/PID/Subsystem6 ==
  e : Inport
  antiw : Inport  Port=2
  Avoid windup : Constant  Value=0
  Clamping : Subsystem
  Derivative Gain : Gain  Gain=Kd
  Filtered Derivative : TransferFcn  Denominator=Tf
  Integral Gain : Gain  Gain=Ki
  Integrator : Integrator
  Proportional Gain : Gain  Gain=Kp
  Sum action : Sum  Inputs=+++
  Switch1 : Switch  Criteria=u2 > Threshold
  u : Outport
  wires:
  Clamping/1(Clamping) -> Switch1/2  "Clamping"
  antiw/1 -> Clamping/2(antiw)  "antiw"
  Integrator/1 -> Sum action/3
  Proportional Gain/1 -> Sum action/1
  Avoid windup/1 -> Switch1/1
  Integral Gain/1 -> Switch1/3
  Switch1/1 -> Integrator/1
  e/1 -> Derivative Gain/1, Integral Gain/1, Clamping/3(e), Proportional Gain/1  "e"
  Derivative Gain/1 -> Filtered Derivative/1
  Sum action/1 -> u/1, Clamping/1(u)  "u"
  Filtered Derivative/1 -> Sum action/2

== system ControlSystem/Variant system/MIMO/Variant Controller/PID/Subsystem7 ==
  e : Inport
  antiw : Inport  Port=2
  Avoid windup : Constant  Value=0
  Clamping : Subsystem
  Derivative Gain : Gain  Gain=Kd
  Filtered Derivative : TransferFcn  Denominator=Tf
  Integral Gain : Gain  Gain=Ki
  Integrator : Integrator
  Proportional Gain : Gain  Gain=Kp
  Sum action : Sum  Inputs=+++
  Switch1 : Switch  Criteria=u2 > Threshold
  u : Outport
  wires:
  Filtered Derivative/1 -> Sum action/2
  Sum action/1 -> Clamping/1(u), u/1  "u"
  Derivative Gain/1 -> Filtered Derivative/1
  e/1 -> Proportional Gain/1, Clamping/3(e), Integral Gain/1, Derivative Gain/1  "e"
  Switch1/1 -> Integrator/1
  Integral Gain/1 -> Switch1/3
  Avoid windup/1 -> Switch1/1
  Proportional Gain/1 -> Sum action/1
  Integrator/1 -> Sum action/3
  antiw/1 -> Clamping/2(antiw)  "antiw"
  Clamping/1(Clamping) -> Switch1/2  "Clamping"

== system ControlSystem/Variant system/MIMO/Variant Controller/PID/Subsystem8 ==
  e : Inport
  antiw : Inport  Port=2
  Avoid windup : Constant  Value=0
  Clamping : Subsystem
  Derivative Gain : Gain  Gain=Kd
  Filtered Derivative : TransferFcn  Denominator=Tf
  Integral Gain : Gain  Gain=Ki
  Integrator : Integrator
  Proportional Gain : Gain  Gain=Kp
  Sum action : Sum  Inputs=+++
  Switch1 : Switch  Criteria=u2 > Threshold
  u : Outport
  wires:
  Clamping/1(Clamping) -> Switch1/2  "Clamping"
  antiw/1 -> Clamping/2(antiw)  "antiw"
  Integrator/1 -> Sum action/3
  Proportional Gain/1 -> Sum action/1
  Avoid windup/1 -> Switch1/1
  Integral Gain/1 -> Switch1/3
  Switch1/1 -> Integrator/1
  e/1 -> Derivative Gain/1, Integral Gain/1, Clamping/3(e), Proportional Gain/1  "e"
  Derivative Gain/1 -> Filtered Derivative/1
  Sum action/1 -> u/1, Clamping/1(u)  "u"
  Filtered Derivative/1 -> Sum action/2

== system ControlSystem/Variant system/MIMO/Variant Controller/PID/Subsystem9 ==
  e : Inport
  antiw : Inport  Port=2
  Avoid windup : Constant  Value=0
  Clamping : Subsystem
  Derivative Gain : Gain  Gain=Kd
  Filtered Derivative : TransferFcn  Denominator=Tf
  Integral Gain : Gain  Gain=Ki
  Integrator : Integrator
  Proportional Gain : Gain  Gain=Kp
  Sum action : Sum  Inputs=+++
  Switch1 : Switch  Criteria=u2 > Threshold
  u : Outport
  wires:
  Filtered Derivative/1 -> Sum action/2
  Sum action/1 -> Clamping/1(u), u/1  "u"
  Derivative Gain/1 -> Filtered Derivative/1
  e/1 -> Proportional Gain/1, Clamping/3(e), Integral Gain/1, Derivative Gain/1  "e"
  Switch1/1 -> Integrator/1
  Integral Gain/1 -> Switch1/3
  Avoid windup/1 -> Switch1/1
  Proportional Gain/1 -> Sum action/1
  Integrator/1 -> Sum action/3
  antiw/1 -> Clamping/2(antiw)  "antiw"
  Clamping/1(Clamping) -> Switch1/2  "Clamping"

== system ControlSystem/Variant system/MIMO/Variant Controller/Rlocusantiwindup/Subsystem1 ==
  e : Inport
  antiw : Inport  Port=2
  Avoid windup : Constant  Value=0
  Clamping : Subsystem
  Integral Gain : Gain  Gain=Ki
  Integrator : Integrator
  Proportional Gain : Gain  Gain=Kp
  Sum action : Sum  Inputs=+++
  Switch1 : Switch  Criteria=u2 > Threshold
  ZPK compensator : cstblocks/LTI System  sys=Compensator  IC=[]
  u : Outport
  wires:
  Sum action/1 -> Clamping/1(u), u/1  "u"
  ZPK compensator/1 -> Sum action/2
  e/1 -> ZPK compensator/1, Proportional Gain/1, Clamping/3(e), Integral Gain/1  "e"
  Switch1/1 -> Integrator/1
  Integral Gain/1 -> Switch1/3
  Avoid windup/1 -> Switch1/1
  Proportional Gain/1 -> Sum action/1
  Integrator/1 -> Sum action/3
  antiw/1 -> Clamping/2(antiw)  "antiw"
  Clamping/1(Clamping) -> Switch1/2  "Clamping"

== system ControlSystem/Variant system/MIMO/Variant Controller/Rlocusantiwindup/Subsystem11 ==
  e : Inport
  antiw : Inport  Port=2
  Avoid windup : Constant  Value=0
  Clamping : Subsystem
  Integral Gain : Gain  Gain=Ki
  Integrator : Integrator
  Proportional Gain : Gain  Gain=Kp
  Sum action : Sum  Inputs=+++
  Switch1 : Switch  Criteria=u2 > Threshold
  ZPK compensator : cstblocks/LTI System  sys=Compensator  IC=[]
  u : Outport
  wires:
  Clamping/1(Clamping) -> Switch1/2  "Clamping"
  antiw/1 -> Clamping/2(antiw)  "antiw"
  Integrator/1 -> Sum action/3
  Proportional Gain/1 -> Sum action/1
  Avoid windup/1 -> Switch1/1
  Integral Gain/1 -> Switch1/3
  Switch1/1 -> Integrator/1
  e/1 -> Integral Gain/1, Clamping/3(e), Proportional Gain/1, ZPK compensator/1  "e"
  ZPK compensator/1 -> Sum action/2
  Sum action/1 -> u/1, Clamping/1(u)  "u"

== system ControlSystem/Variant system/MIMO/Variant Controller/Rlocusantiwindup/Subsystem12 ==
  e : Inport
  antiw : Inport  Port=2
  Avoid windup : Constant  Value=0
  Clamping : Subsystem
  Integral Gain : Gain  Gain=Ki
  Integrator : Integrator
  Proportional Gain : Gain  Gain=Kp
  Sum action : Sum  Inputs=+++
  Switch1 : Switch  Criteria=u2 > Threshold
  ZPK compensator : cstblocks/LTI System  sys=Compensator  IC=[]
  u : Outport
  wires:
  Clamping/1(Clamping) -> Switch1/2  "Clamping"
  antiw/1 -> Clamping/2(antiw)  "antiw"
  Integrator/1 -> Sum action/3
  Proportional Gain/1 -> Sum action/1
  Avoid windup/1 -> Switch1/1
  Integral Gain/1 -> Switch1/3
  Switch1/1 -> Integrator/1
  e/1 -> Integral Gain/1, Clamping/3(e), Proportional Gain/1, ZPK compensator/1  "e"
  ZPK compensator/1 -> Sum action/2
  Sum action/1 -> u/1, Clamping/1(u)  "u"

== system ControlSystem/Variant system/MIMO/Variant Controller/Rlocusantiwindup/Subsystem15 ==
  e : Inport
  antiw : Inport  Port=2
  Avoid windup : Constant  Value=0
  Clamping : Subsystem
  Integral Gain : Gain  Gain=Ki
  Integrator : Integrator
  Proportional Gain : Gain  Gain=Kp
  Sum action : Sum  Inputs=+++
  Switch1 : Switch  Criteria=u2 > Threshold
  ZPK compensator : cstblocks/LTI System  sys=Compensator  IC=[]
  u : Outport
  wires:
  Sum action/1 -> Clamping/1(u), u/1  "u"
  ZPK compensator/1 -> Sum action/2
  e/1 -> ZPK compensator/1, Proportional Gain/1, Clamping/3(e), Integral Gain/1  "e"
  Switch1/1 -> Integrator/1
  Integral Gain/1 -> Switch1/3
  Avoid windup/1 -> Switch1/1
  Proportional Gain/1 -> Sum action/1
  Integrator/1 -> Sum action/3
  antiw/1 -> Clamping/2(antiw)  "antiw"
  Clamping/1(Clamping) -> Switch1/2  "Clamping"

== system ControlSystem/Variant system/MIMO/Variant Controller/Rlocusantiwindup/Subsystem2 ==
  e : Inport
  antiw : Inport  Port=2
  Avoid windup : Constant  Value=0
  Clamping : Subsystem
  Integral Gain : Gain  Gain=Ki
  Integrator : Integrator
  Proportional Gain : Gain  Gain=Kp
  Sum action : Sum  Inputs=+++
  Switch1 : Switch  Criteria=u2 > Threshold
  ZPK compensator : cstblocks/LTI System  sys=Compensator  IC=[]
  u : Outport
  wires:
  Sum action/1 -> Clamping/1(u), u/1  "u"
  ZPK compensator/1 -> Sum action/2
  e/1 -> ZPK compensator/1, Proportional Gain/1, Clamping/3(e), Integral Gain/1  "e"
  Switch1/1 -> Integrator/1
  Integral Gain/1 -> Switch1/3
  Avoid windup/1 -> Switch1/1
  Proportional Gain/1 -> Sum action/1
  Integrator/1 -> Sum action/3
  antiw/1 -> Clamping/2(antiw)  "antiw"
  Clamping/1(Clamping) -> Switch1/2  "Clamping"

== system ControlSystem/Variant system/MIMO/Variant Controller/Rlocusantiwindup/Subsystem3 ==
  e : Inport
  antiw : Inport  Port=2
  Avoid windup : Constant  Value=0
  Clamping : Subsystem
  Integral Gain : Gain  Gain=Ki
  Integrator : Integrator
  Proportional Gain : Gain  Gain=Kp
  Sum action : Sum  Inputs=+++
  Switch1 : Switch  Criteria=u2 > Threshold
  ZPK compensator : cstblocks/LTI System  sys=Compensator  IC=[]
  u : Outport
  wires:
  Clamping/1(Clamping) -> Switch1/2  "Clamping"
  antiw/1 -> Clamping/2(antiw)  "antiw"
  Integrator/1 -> Sum action/3
  Proportional Gain/1 -> Sum action/1
  Avoid windup/1 -> Switch1/1
  Integral Gain/1 -> Switch1/3
  Switch1/1 -> Integrator/1
  e/1 -> Integral Gain/1, Clamping/3(e), Proportional Gain/1, ZPK compensator/1  "e"
  ZPK compensator/1 -> Sum action/2
  Sum action/1 -> u/1, Clamping/1(u)  "u"

== system ControlSystem/Variant system/MIMO/Variant Controller/Rlocusantiwindup/Subsystem4 ==
  e : Inport
  antiw : Inport  Port=2
  Avoid windup : Constant  Value=0
  Clamping : Subsystem
  Integral Gain : Gain  Gain=Ki
  Integrator : Integrator
  Proportional Gain : Gain  Gain=Kp
  Sum action : Sum  Inputs=+++
  Switch1 : Switch  Criteria=u2 > Threshold
  ZPK compensator : cstblocks/LTI System  sys=Compensator  IC=[]
  u : Outport
  wires:
  Sum action/1 -> Clamping/1(u), u/1  "u"
  ZPK compensator/1 -> Sum action/2
  e/1 -> ZPK compensator/1, Proportional Gain/1, Clamping/3(e), Integral Gain/1  "e"
  Switch1/1 -> Integrator/1
  Integral Gain/1 -> Switch1/3
  Avoid windup/1 -> Switch1/1
  Proportional Gain/1 -> Sum action/1
  Integrator/1 -> Sum action/3
  antiw/1 -> Clamping/2(antiw)  "antiw"
  Clamping/1(Clamping) -> Switch1/2  "Clamping"

== system ControlSystem/Variant system/MIMO/Variant Controller/Rlocusantiwindup/Subsystem5 ==
  e : Inport
  antiw : Inport  Port=2
  Avoid windup : Constant  Value=0
  Clamping : Subsystem
  Integral Gain : Gain  Gain=Ki
  Integrator : Integrator
  Proportional Gain : Gain  Gain=Kp
  Sum action : Sum  Inputs=+++
  Switch1 : Switch  Criteria=u2 > Threshold
  ZPK compensator : cstblocks/LTI System  sys=Compensator  IC=[]
  u : Outport
  wires:
  Clamping/1(Clamping) -> Switch1/2  "Clamping"
  antiw/1 -> Clamping/2(antiw)  "antiw"
  Integrator/1 -> Sum action/3
  Proportional Gain/1 -> Sum action/1
  Avoid windup/1 -> Switch1/1
  Integral Gain/1 -> Switch1/3
  Switch1/1 -> Integrator/1
  e/1 -> Integral Gain/1, Clamping/3(e), Proportional Gain/1, ZPK compensator/1  "e"
  ZPK compensator/1 -> Sum action/2
  Sum action/1 -> u/1, Clamping/1(u)  "u"

== system ControlSystem/Variant system/MIMO/Variant Controller/Rlocusantiwindup/Subsystem6 ==
  e : Inport
  antiw : Inport  Port=2
  Avoid windup : Constant  Value=0
  Clamping : Subsystem
  Integral Gain : Gain  Gain=Ki
  Integrator : Integrator
  Proportional Gain : Gain  Gain=Kp
  Sum action : Sum  Inputs=+++
  Switch1 : Switch  Criteria=u2 > Threshold
  ZPK compensator : cstblocks/LTI System  sys=Compensator  IC=[]
  u : Outport
  wires:
  Sum action/1 -> Clamping/1(u), u/1  "u"
  ZPK compensator/1 -> Sum action/2
  e/1 -> ZPK compensator/1, Proportional Gain/1, Clamping/3(e), Integral Gain/1  "e"
  Switch1/1 -> Integrator/1
  Integral Gain/1 -> Switch1/3
  Avoid windup/1 -> Switch1/1
  Proportional Gain/1 -> Sum action/1
  Integrator/1 -> Sum action/3
  antiw/1 -> Clamping/2(antiw)  "antiw"
  Clamping/1(Clamping) -> Switch1/2  "Clamping"

== system ControlSystem/Variant system/MIMO/Variant Controller/Rlocusantiwindup/Subsystem7 ==
  e : Inport
  antiw : Inport  Port=2
  Avoid windup : Constant  Value=0
  Clamping : Subsystem
  Integral Gain : Gain  Gain=Ki
  Integrator : Integrator
  Proportional Gain : Gain  Gain=Kp
  Sum action : Sum  Inputs=+++
  Switch1 : Switch  Criteria=u2 > Threshold
  ZPK compensator : cstblocks/LTI System  sys=Compensator  IC=[]
  u : Outport
  wires:
  Clamping/1(Clamping) -> Switch1/2  "Clamping"
  antiw/1 -> Clamping/2(antiw)  "antiw"
  Integrator/1 -> Sum action/3
  Proportional Gain/1 -> Sum action/1
  Avoid windup/1 -> Switch1/1
  Integral Gain/1 -> Switch1/3
  Switch1/1 -> Integrator/1
  e/1 -> Integral Gain/1, Clamping/3(e), Proportional Gain/1, ZPK compensator/1  "e"
  ZPK compensator/1 -> Sum action/2
  Sum action/1 -> u/1, Clamping/1(u)  "u"

== system ControlSystem/Variant system/MIMO/Variant Controller/Rlocusantiwindup/Subsystem8 ==
  e : Inport
  antiw : Inport  Port=2
  Avoid windup : Constant  Value=0
  Clamping : Subsystem
  Integral Gain : Gain  Gain=Ki
  Integrator : Integrator
  Proportional Gain : Gain  Gain=Kp
  Sum action : Sum  Inputs=+++
  Switch1 : Switch  Criteria=u2 > Threshold
  ZPK compensator : cstblocks/LTI System  sys=Compensator  IC=[]
  u : Outport
  wires:
  Sum action/1 -> Clamping/1(u), u/1  "u"
  ZPK compensator/1 -> Sum action/2
  e/1 -> ZPK compensator/1, Proportional Gain/1, Clamping/3(e), Integral Gain/1  "e"
  Switch1/1 -> Integrator/1
  Integral Gain/1 -> Switch1/3
  Avoid windup/1 -> Switch1/1
  Proportional Gain/1 -> Sum action/1
  Integrator/1 -> Sum action/3
  antiw/1 -> Clamping/2(antiw)  "antiw"
  Clamping/1(Clamping) -> Switch1/2  "Clamping"

== system ControlSystem/Variant system/MIMO/Variant Controller/Rlocusantiwindup/Subsystem9 ==
  e : Inport
  antiw : Inport  Port=2
  Avoid windup : Constant  Value=0
  Clamping : Subsystem
  Integral Gain : Gain  Gain=Ki
  Integrator : Integrator
  Proportional Gain : Gain  Gain=Kp
  Sum action : Sum  Inputs=+++
  Switch1 : Switch  Criteria=u2 > Threshold
  ZPK compensator : cstblocks/LTI System  sys=Compensator  IC=[]
  u : Outport
  wires:
  Clamping/1(Clamping) -> Switch1/2  "Clamping"
  antiw/1 -> Clamping/2(antiw)  "antiw"
  Integrator/1 -> Sum action/3
  Proportional Gain/1 -> Sum action/1
  Avoid windup/1 -> Switch1/1
  Integral Gain/1 -> Switch1/3
  Switch1/1 -> Integrator/1
  e/1 -> Integral Gain/1, Clamping/3(e), Proportional Gain/1, ZPK compensator/1  "e"
  ZPK compensator/1 -> Sum action/2
  Sum action/1 -> u/1, Clamping/1(u)  "u"

== system ControlSystem/Variant system/SISO/Variant Controller/PID/Subsystem1 ==
  e : Inport
  antiw : Inport  Port=2
  Avoid windup : Constant  Value=0
  Clamping : Subsystem
  Derivative Gain : Gain  Gain=Kd
  Filtered Derivative : TransferFcn  Denominator=Tf
  Integral Gain : Gain  Gain=Ki
  Integrator : Integrator
  Proportional Gain : Gain  Gain=Kp
  Sum action : Sum  Inputs=+++
  Switch1 : Switch  Criteria=u2 > Threshold
  u : Outport
  wires:
  Clamping/1(Clamping) -> Switch1/2  "Clamping"
  antiw/1 -> Clamping/2(antiw)  "antiw"
  Integrator/1 -> Sum action/3
  Proportional Gain/1 -> Sum action/1
  Avoid windup/1 -> Switch1/1
  Integral Gain/1 -> Switch1/3
  Switch1/1 -> Integrator/1
  e/1 -> Derivative Gain/1, Integral Gain/1, Clamping/3(e), Proportional Gain/1  "e"
  Derivative Gain/1 -> Filtered Derivative/1
  Sum action/1 -> u/1, Clamping/1(u)  "u"
  Filtered Derivative/1 -> Sum action/2

== system ControlSystem/Variant system/SISO/Variant Controller/PID/Subsystem10 ==
  e : Inport
  antiw : Inport  Port=2
  Avoid windup : Constant  Value=0
  Clamping : Subsystem
  Derivative Gain : Gain  Gain=Kd
  Filtered Derivative : TransferFcn  Denominator=Tf
  Integral Gain : Gain  Gain=Ki
  Integrator : Integrator
  Proportional Gain : Gain  Gain=Kp
  Sum action : Sum  Inputs=+++
  Switch1 : Switch  Criteria=u2 > Threshold
  u : Outport
  wires:
  Clamping/1(Clamping) -> Switch1/2  "Clamping"
  antiw/1 -> Clamping/2(antiw)  "antiw"
  Integrator/1 -> Sum action/3
  Proportional Gain/1 -> Sum action/1
  Avoid windup/1 -> Switch1/1
  Integral Gain/1 -> Switch1/3
  Switch1/1 -> Integrator/1
  e/1 -> Derivative Gain/1, Integral Gain/1, Clamping/3(e), Proportional Gain/1  "e"
  Derivative Gain/1 -> Filtered Derivative/1
  Sum action/1 -> u/1, Clamping/1(u)  "u"
  Filtered Derivative/1 -> Sum action/2

== system ControlSystem/Variant system/SISO/Variant Controller/PID/Subsystem11 ==
  e : Inport
  antiw : Inport  Port=2
  Avoid windup : Constant  Value=0
  Clamping : Subsystem
  Derivative Gain : Gain  Gain=Kd
  Filtered Derivative : TransferFcn  Denominator=Tf
  Integral Gain : Gain  Gain=Ki
  Integrator : Integrator
  Proportional Gain : Gain  Gain=Kp
  Sum action : Sum  Inputs=+++
  Switch1 : Switch  Criteria=u2 > Threshold
  u : Outport
  wires:
  Filtered Derivative/1 -> Sum action/2
  Sum action/1 -> Clamping/1(u), u/1  "u"
  Derivative Gain/1 -> Filtered Derivative/1
  e/1 -> Proportional Gain/1, Clamping/3(e), Integral Gain/1, Derivative Gain/1  "e"
  Switch1/1 -> Integrator/1
  Integral Gain/1 -> Switch1/3
  Avoid windup/1 -> Switch1/1
  Proportional Gain/1 -> Sum action/1
  Integrator/1 -> Sum action/3
  antiw/1 -> Clamping/2(antiw)  "antiw"
  Clamping/1(Clamping) -> Switch1/2  "Clamping"
